simulink model "hcs_test"  (R2018a)
settings: Solver=VariableStepAuto  StartTime=0.0  StopTime=33  RelTol=1e-3
settings Model: Creator=BEAR  LastModifiedBy=BEAR

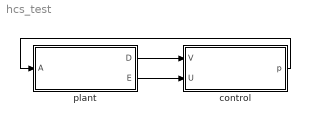
== system hcs_test ==
  control : Subsystem
  plant : Subsystem
  wires:
  control/1(p) -> plant/1(A)
  plant/2(E) -> control/2(U)
  plant/1(D) -> control/1(V)

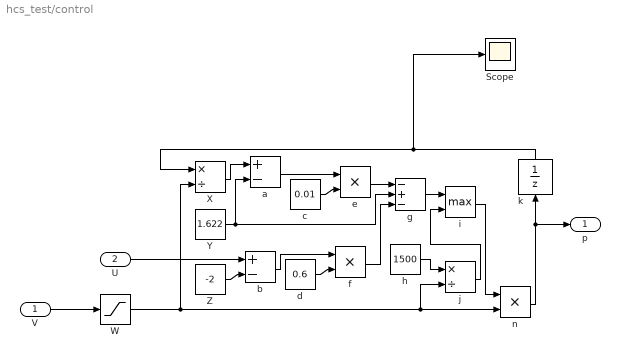
== system hcs_test/control ==
  V : Inport
  U : Inport  Port=2
  Scope : Scope
  W : Saturate  UpperLimit=800  LowerLimit=600
  X : Product  Inputs=*/  SampleTime=0.128
  Y : Constant  Value=1.622
  Z : Constant  Value=-2
  a : Sum  Inputs=+-  SampleTime=0.128
  b : Sum  Inputs=+-  SampleTime=0.128
  c : Constant  Value=0.01
  d : Constant  Value=0.6
  e : Product  Inputs=**  SampleTime=0.128
  f : Product  Inputs=**  SampleTime=0.128
  g : Sum  Inputs=-+-  SampleTime=0.128
  h : Constant  Value=1500
  i : MinMax  Function=max  Inputs=2  SampleTime=0.128
  j : Product  Inputs=*/  SampleTime=0.128
  k : UnitDelay  InitialCondition=2027.5  SampleTime=0.128
  n : Product  Inputs=**  SampleTime=0.128
  p : Outport
  wires:
  X/1 -> a/1
  Y/1 -> g/2, a/2
  a/1 -> e/1
  c/1 -> e/2
  Z/1 -> b/2
  b/1 -> f/1
  d/1 -> f/2
  f/1 -> g/3
  U/1 -> b/1
  g/1 -> i/1
  k/1 -> Scope/1, X/1
  e/1 -> g/1
  W/1 -> X/2, n/2, j/2
  n/1 -> k/1, p/1
  i/1 -> n/1
  h/1 -> j/1
  j/1 -> i/2
  V/1 -> W/1

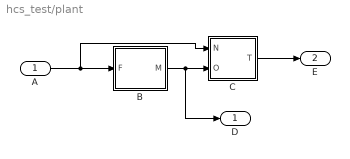
== system hcs_test/plant ==
  A : Inport
  B : Subsystem
  C : Subsystem
  D : Outport
  E : Outport  Port=2
  wires:
  B/1(M) -> C/2(O), D/1
  C/1(T) -> E/1
  A/1 -> C/1(N), B/1(F)

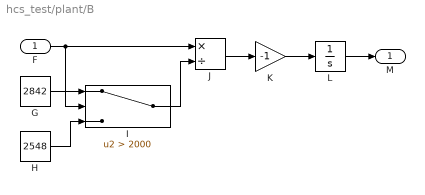
== system hcs_test/plant/B ==
  F : Inport
  G : Constant  Value=2842
  H : Constant  Value=2548
  I : Switch  Criteria=u2 > Threshold  Threshold=2000  SampleTime=0
  J : Product  Inputs=*/  SampleTime=0
  K : Gain  Gain=-1  SampleTime=0
  L : Integrator  InitialCondition=1250
  M : Outport
  wires:
  F/1 -> J/1, I/2
  J/1 -> K/1
  K/1 -> L/1
  L/1 -> M/1
  G/1 -> I/1
  H/1 -> I/3
  I/1 -> J/2

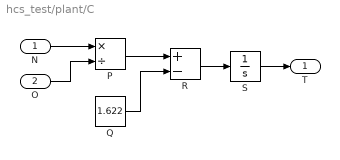
== system hcs_test/plant/C ==
  N : Inport
  O : Inport  Port=2
  P : Product  Inputs=*/  SampleTime=0
  Q : Constant  Value=1.622
  R : Sum  Inputs=+-  SampleTime=0
  S : Integrator  InitialCondition=-2
  T : Outport
  wires:
  N/1 -> P/1
  O/1 -> P/2
  P/1 -> R/1
  Q/1 -> R/2
  R/1 -> S/1
  S/1 -> T/1
